simulink model "pospolix_4gdl_discretizzatoslx"  (R2021a)
settings: Solver=VariableStepAuto  StartTime=0.0  StopTime=1.5  RelTol=1e-3
values from neighbouring files (symbols this model uses):
  m = config_dc(parx)    [main.m]
  parx = parametri()    [main.m]
  pp_c = pos_poli_cc_x(m, ac,2)    [main.m]
  pp_m = pos_poli_cc_x(m, ac,1)    [main.m]
undefined symbols (not defined in the file or in its folder): accelerazioni, Evaluate_Trajectory
libraries: simulink x2
settings Model: Creator=user  LastModifiedBy=stefa
settings SolverCC: AlgebraicLoopSolver=TrustRegion
settings DebuggingCC: SFMachineParentedDataDiag=warning

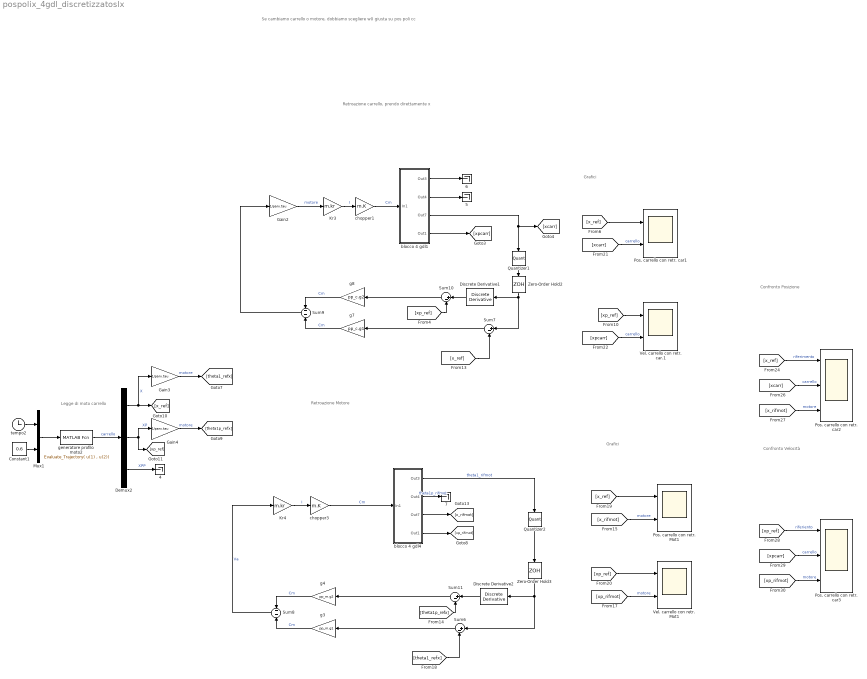
== system pospolix_4gdl_discretizzatoslx ==
  note: Se cambiamo carrello o motore, dobbiamo scegliere w0 giusta su pos poli cc
  note: Confronto
      | Velocità
  note: Confronto Posizione
  note: Grafici
  note: Retroazione Motore
  note: Retroazione carrello, prendo direttamente x
  note: Grafici
  note: Legge di moto carrello
   {4..7} (4 alike) : Terminator
  Constant1 : Constant  Value=0.6
  Demux2 : Demux  Outputs=3
  Discrete Derivative1 : simulink/Discrete/Discrete Derivative  gainval=1.0  ICPrevScaledInput=0.0  OutMin=[]  OutMax=[]  OutDataType=fixdt(1, 16)  OutScaling=2^-10  DoSatur=off
  Discrete Derivative2 : simulink/Discrete/Discrete Derivative  gainval=1.0  ICPrevScaledInput=0.0  OutMin=[]  OutMax=[]  OutDataType=fixdt(1, 16)  OutScaling=2^-10  DoSatur=off
  Gain2 : Gain  Gain=1/parx.tau
  Gain3 : Gain  Gain=1/parx.tau
  Gain4 : Gain  Gain=1/parx.tau
  Kr3 : Gain  Gain=m.kr
  Kr4 : Gain  Gain=m.kr
  Mux1 : Mux  Inputs=2
  Pos. carrello con retr. Mot1 : Scope  NumInputPorts=2
  Pos. carrello con retr. car1 : Scope  NumInputPorts=2
  Pos. carrello con retr. car2 : Scope  NumInputPorts=3
  Pos. carrello con retr. car3 : Scope  NumInputPorts=3
  Quantizer1 : Quantizer  QuantizationInterval=10/4096
  Quantizer2 : Quantizer  QuantizationInterval=10/4096
  Sum{6..7,10..11} (4 alike) : Sum  Inputs=|+-
  Sum8 : Sum  Inputs=--
  Sum9 : Sum  Inputs=--
  Vel. carrello con retr. Mot1 : Scope  NumInputPorts=2
  Vel. carrello con retr. car.1 : Scope  NumInputPorts=2
  Zero-Order Hold2 : ZeroOrderHold  SampleTime=0.001
  Zero-Order Hold3 : ZeroOrderHold  SampleTime=0.001
  blocco 4 gdl1 : Subsystem
  blocco 4 gdl4 : Subsystem
  chopper1 : Gain  Gain=m.K
  chopper3 : Gain  Gain=m.K
  g3 : Gain  Gain=pp_m.g1
  g4 : Gain  Gain=pp_m.g2
  g7 : Gain  Gain=pp_c.g1
  g8 : Gain  Gain=pp_c.g2
  generatore profilo moto2 : MATLABFcn  MATLABFcn=Evaluate_Trajectory( u(1) , u(2))  OutputDimensions=3
  tempo2 : Clock
  wires:
  Gain4/1 -> [theta1p_refx]  "motore"
  [xpcarr] -> Vel. carrello con retr. car.1/2  "carrello"
  [x_ref] -> Pos. carrello con retr. car2/1  "riferimento"
  [xp_rifmot] -> Pos. carrello con retr. car3/3  "motore"
  [xp_ref] -> Pos. carrello con retr. car3/1  "riferiento"
  [x_rifmot] -> Pos. carrello con retr. car2/3  "motore"
  [xpcarr] -> Pos. carrello con retr. car3/2  "carrello"
  Demux2/2 -> Gain4/1, [xp_ref]  "XP"
  chopper3/1 -> blocco 4 gdl4/1(In1)  "Cm"
  generatore profilo moto2/1 -> Demux2/1  "carrello"
  Sum6/1 -> g3/1
  blocco 4 gdl4/4(Out1) -> [xp_rifmot]
  Demux2/1 -> [x_ref], Gain3/1  "X"
  Kr4/1 -> chopper3/1  "I"
  Gain3/1 -> [theta1_refx]  "motore"
  [x_ref] -> Sum7/2
  [x_ref] -> Pos. carrello con retr. Mot1/1
  [theta1_refx] -> Sum6/2
  Kr3/1 -> chopper1/1  "I"
  [xp_ref] -> Vel. carrello con retr. Mot1/1
  [xcarr] -> Pos. carrello con retr. car2/2  "carrello"
  [xp_ref] -> Vel. carrello con retr. car.1/1
  Sum11/1 -> g4/1
  blocco 4 gdl1/1(Out3) -> " 6"/1
  Demux2/3 -> " 4"/1  "XPP"
  g8/1 -> Sum9/1  "Cm"
  g4/1 -> Sum8/1  "Cm"
  [xp_ref] -> Sum10/2
  Sum9/1 -> Gain2/1
  Gain2/1 -> Kr3/1  "motore"
  chopper1/1 -> blocco 4 gdl1/1(In1)  "Cm"
  Sum7/1 -> g7/1
  blocco 4 gdl1/2(Out4) -> " 5"/1
  blocco 4 gdl1/3(Out7) -> [xcarr], Quantizer1/1
  blocco 4 gdl4/3(Out7) -> [x_rifmot]
  g7/1 -> Sum9/2  "Cm"
  [xp_rifmot] -> Vel. carrello con retr. Mot1/2  "motore"
  Sum8/1 -> Kr4/1  "Va"
  blocco 4 gdl1/4(Out1) -> [xpcarr]
  Sum10/1 -> g8/1
  g3/1 -> Sum8/2  "Cm"
  [theta1p_refx] -> Sum11/2
  tempo2/1 -> Mux1/1
  Mux1/1 -> generatore profilo moto2/1
  Constant1/1 -> Mux1/2
  [x_ref] -> Pos. carrello con retr. car1/1
  [xcarr] -> Pos. carrello con retr. car1/2  "carrello"
  [x_rifmot] -> Pos. carrello con retr. Mot1/2  "motore"
  Quantizer1/1 -> Zero-Order Hold2/1
  Zero-Order Hold2/1 -> Sum7/1, Discrete Derivative1/1
  Discrete Derivative1/1 -> Sum10/1
  blocco 4 gdl4/1(Out3) -> Quantizer2/1  "theta1_rifmot"
  Quantizer2/1 -> Zero-Order Hold3/1
  Zero-Order Hold3/1 -> Discrete Derivative2/1, Sum6/1
  Discrete Derivative2/1 -> Sum11/1
  blocco 4 gdl4/2(Out4) -> " 7"/1  "theta1p_rifmot"

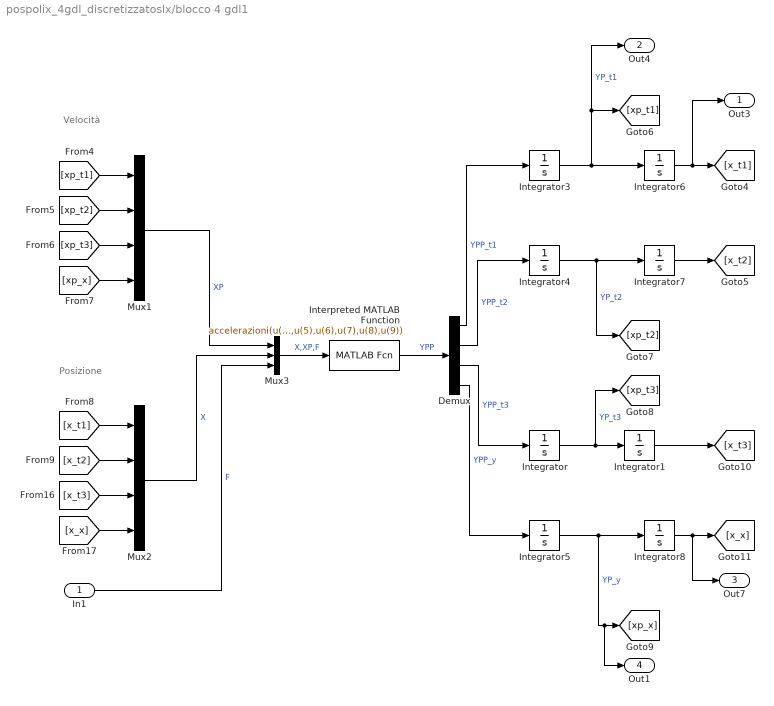
== system pospolix_4gdl_discretizzatoslx/blocco 4 gdl1 ==
  note: Posizione
  note: Velocità
  In1 : Inport
  Demux : Demux
  Integrator{,1,3..7} (7 alike) : Integrator
  Integrator8 : Integrator  InitialCondition=0.0005
  Interpreted MATLAB Function : MATLABFcn  MATLABFcn=accelerazioni(u(1),u(2),u(3),u(4),u(5),u(6),u(7),u(8),u(9))  OutputDimensions=4
  Mux1 : Mux
  Mux2 : Mux
  Mux3 : Mux  Inputs=3
  Out3 : Outport
  Out4 : Outport  Port=2
  Out7 : Outport  Port=3
  Out1 : Outport  Port=4
  wires:
  [xp_t3] -> Mux1/3
  Interpreted MATLAB Function/1 -> Demux/1  "YPP"
  Integrator3/1 -> Out4/1, [xp_t1], Integrator6/1  "YP_t1"
  Integrator8/1 -> Out7/1, [x_x]
  Integrator7/1 -> [x_t2]
  [xp_x] -> Mux1/4
  [x_t1] -> Mux2/1
  Mux1/1 -> Mux3/1  "XP"
  [x_x] -> Mux2/4
  Demux/3 -> Integrator/1  "YPP_t3"
  Integrator/1 -> Integrator1/1, [xp_t3]  "YP_t3"
  Mux2/1 -> Mux3/2  "X"
  Integrator6/1 -> Out3/1, [x_t1]
  Integrator5/1 -> Out1/1, [xp_x], Integrator8/1  "YP_y"
  [xp_t2] -> Mux1/2
  Mux3/1 -> Interpreted MATLAB Function/1  "X,XP,F"
  [x_t3] -> Mux2/3
  In1/1 -> Mux3/3  "F"
  Demux/4 -> Integrator5/1  "YPP_y"
  Integrator4/1 -> [xp_t2], Integrator7/1  "YP_t2"
  Integrator1/1 -> [x_t3]
  [xp_t1] -> Mux1/1
  [x_t2] -> Mux2/2
  Demux/2 -> Integrator4/1  "YPP_t2"
  Demux/1 -> Integrator3/1  "YPP_t1"

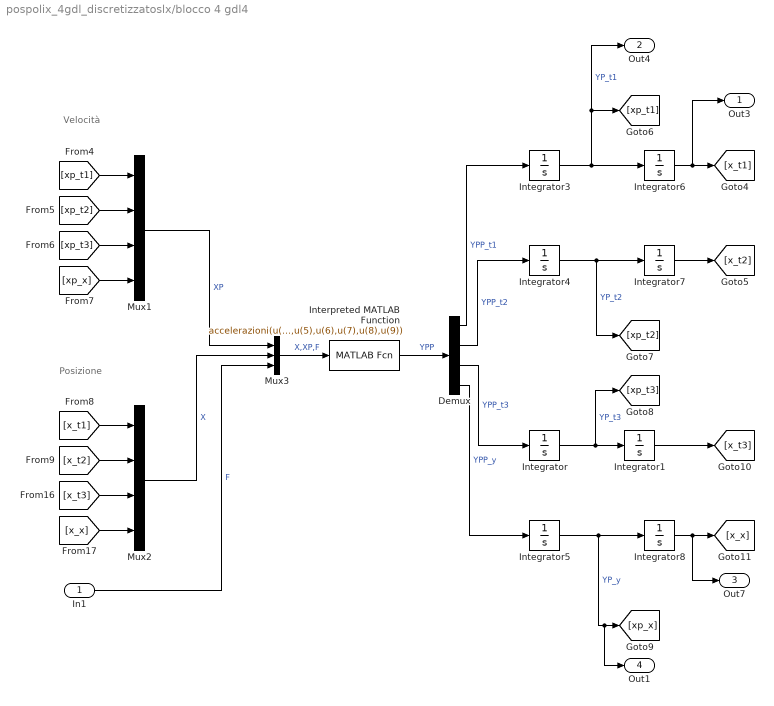
== system pospolix_4gdl_discretizzatoslx/blocco 4 gdl4 ==
  note: Posizione
  note: Velocità
  In1 : Inport
  Demux : Demux
  Integrator{,1,3..7} (7 alike) : Integrator
  Integrator8 : Integrator  InitialCondition=0.0005
  Interpreted MATLAB Function : MATLABFcn  MATLABFcn=accelerazioni(u(1),u(2),u(3),u(4),u(5),u(6),u(7),u(8),u(9))  OutputDimensions=4
  Mux1 : Mux
  Mux2 : Mux
  Mux3 : Mux  Inputs=3
  Out3 : Outport
  Out4 : Outport  Port=2
  Out7 : Outport  Port=3
  Out1 : Outport  Port=4
  wires:
  [xp_t3] -> Mux1/3
  Interpreted MATLAB Function/1 -> Demux/1  "YPP"
  Integrator3/1 -> Out4/1, [xp_t1], Integrator6/1  "YP_t1"
  Integrator8/1 -> Out7/1, [x_x]
  Integrator7/1 -> [x_t2]
  [xp_x] -> Mux1/4
  [x_t1] -> Mux2/1
  Mux1/1 -> Mux3/1  "XP"
  [x_x] -> Mux2/4
  Demux/3 -> Integrator/1  "YPP_t3"
  Integrator/1 -> Integrator1/1, [xp_t3]  "YP_t3"
  Mux2/1 -> Mux3/2  "X"
  Integrator6/1 -> Out3/1, [x_t1]
  Integrator5/1 -> Out1/1, [xp_x], Integrator8/1  "YP_y"
  [xp_t2] -> Mux1/2
  Mux3/1 -> Interpreted MATLAB Function/1  "X,XP,F"
  [x_t3] -> Mux2/3
  In1/1 -> Mux3/3  "F"
  Demux/4 -> Integrator5/1  "YPP_y"
  Integrator4/1 -> [xp_t2], Integrator7/1  "YP_t2"
  Integrator1/1 -> [x_t3]
  [xp_t1] -> Mux1/1
  [x_t2] -> Mux2/2
  Demux/2 -> Integrator4/1  "YPP_t2"
  Demux/1 -> Integrator3/1  "YPP_t1"
